simulink model "simulation_window_3_simulink"  (R2022b)
settings: Solver=VariableStepAuto  StartTime=0.0  StopTime=10.0  RelTol=1e-3
settings Model: Creator=User  LastModifiedBy=User

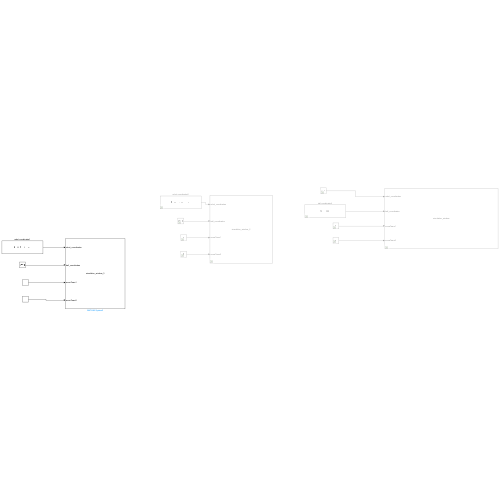
[thumbnail: Simulink's stored preview of the top-level diagram]
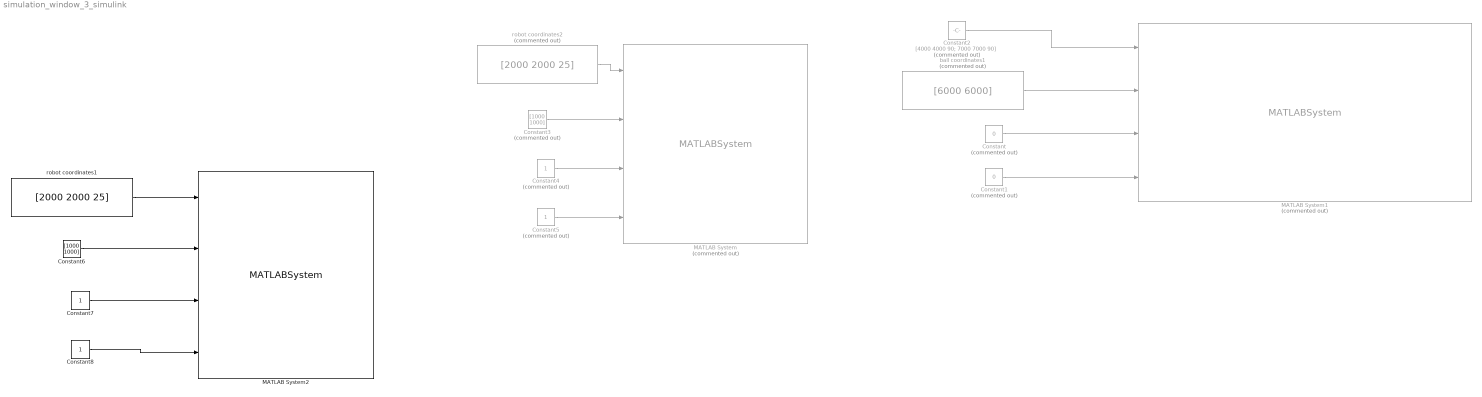
== system simulation_window_3_simulink ==
  Constant : Constant  Commented=on  Value=0
  Constant1 : Constant  Commented=on  Value=0
  Constant2 : Constant  Commented=on  Value=[4000 4000 90; 7000 7000 90]
  Constant3 : Constant  Commented=on  Value=[1000 1000]
  Constant4 : Constant  Commented=on
  Constant5 : Constant  Commented=on
  Constant6 : Constant  Value=[1000 1000]
  Constant7 : Constant
  Constant8 : Constant
  MATLAB System : MATLABSystem  Commented=on  System=simulation_window_2  pitch_length=9000  pitch_width=6000  centre_circle_diameter=1500  border_strip_width=1000  goal_area_length=1000  goal_area_width=1000  penalty_area_length=1000  penalty_area_width=3000  goal_width=2600  goal_depth=500  SimulateUsing=Code generation
      mask Type: simulation_window_2
      mask Display:
      | disp('simulation_window_2');
      | port_label('input',1,'robot_coordinates');
      | port_label('input',2,'ball_coordinates');
      | port_label('input',3,'scoreTeam1');
      | port_label('input',4,'scoreTeam2');
  MATLAB System1 : MATLABSystem  Commented=on  System=simulation_window  pitch_length=9000  pitch_width=6000  centre_circle_diameter=1500  border_strip_width=1000  goal_area_length=1000  goal_area_width=1000  penalty_area_length=1000  penalty_area_width=3000  goal_width=1000  goal_depth=500  SimulateUsing=Code generation
      mask Type: simulation_window
      mask Display:
      | disp('simulation_window');
      | port_label('input',1,'robot_coordinates');
      | port_label('input',2,'ball_coordinates');
      | port_label('input',3,'scoreTeam1');
      | port_label('input',4,'scoreTeam2');
  MATLAB System2 : MATLABSystem  System=simulation_window_3  pitch_length=[]  pitch_width=[]  centre_circle_diameter=[]  border_strip_width=[]  goal_area_length=[]  goal_area_width=[]  penalty_area_length=[]  penalty_area_width=[]  goal_width=[]  goal_depth=[]  SimulateUsing=Code generation
      mask Type: simulation_window_3
      mask Display:
      | disp('simulation_window_3');
      | port_label('input',1,'robot_coordinates');
      | port_label('input',2,'ball_coordinates');
      | port_label('input',3,'scoreTeam1');
      | port_label('input',4,'scoreTeam2');
  ball coordinates1 : Constant  Commented=on  Value=[6000 6000]  VectorParams1D=off
  robot coordinates1 : Constant  Value=[2000 2000 25]  VectorParams1D=off
  robot coordinates2 : Constant  Commented=on  Value=[2000 2000 25]  VectorParams1D=off
  wires:
  Constant/1 -> MATLAB System1/3
  ball coordinates1/1 -> MATLAB System1/2
  Constant1/1 -> MATLAB System1/4
  Constant2/1 -> MATLAB System1/1
  robot coordinates2/1 -> MATLAB System/1
  Constant4/1 -> MATLAB System/3
  Constant5/1 -> MATLAB System/4
  Constant3/1 -> MATLAB System/2
  robot coordinates1/1 -> MATLAB System2/1
  Constant6/1 -> MATLAB System2/2
  Constant7/1 -> MATLAB System2/3
  Constant8/1 -> MATLAB System2/4
